simulink model "PenduloDoblesimulink"  (R2024a)
settings: Solver=VariableStepAuto  StartTime=0.0  StopTime=10.0  RelTol=1e-3
settings Model: Creator=hmax6  LastModifiedBy=100117273
settings RTWCC: GPUComputeCapability=3.5

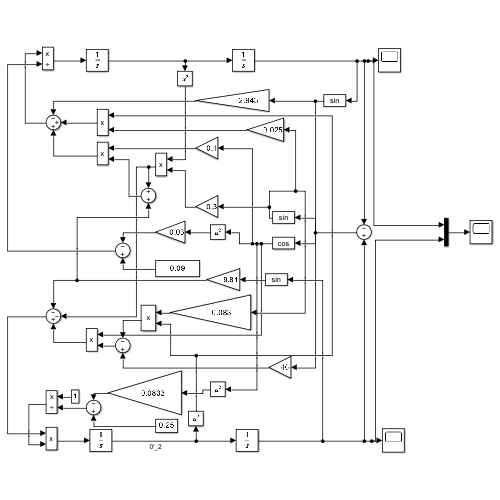
[thumbnail: Simulink's stored preview of the top-level diagram]
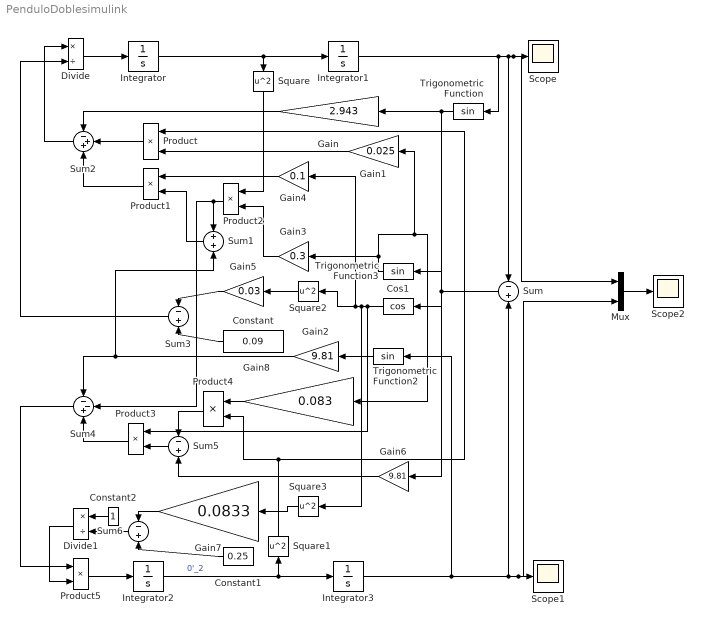
== system PenduloDoblesimulink ==
  Constant : Constant  Value=0.09
  Constant1 : Constant  Value=0.25
  Constant2 : Constant
  Cos1 : Trigonometry  Operator=cos
  Divide : Product  Inputs=*/
  Divide1 : Product  Inputs=*/
  Gain : Gain  Gain=2.943
  Gain1 : Gain  Gain=0.025
  Gain2 : Gain  Gain=9.81
  Gain3 : Gain  Gain=0.3
  Gain4 : Gain  Gain=0.1
  Gain5 : Gain  Gain=0.03
  Gain6 : Gain  Gain=9.81
  Gain7 : Gain  Gain=0.0833
  Gain8 : Gain  Gain=0.083
  Integrator : Integrator
  Integrator1 : Integrator
  Integrator2 : Integrator
  Integrator3 : Integrator  InitialCondition=0.35
  Mux : Mux  Inputs=2
  Product{,1..5} (6 alike) : Product
  Scope : Scope
  Scope1 : Scope
  Scope2 : Scope
  Square{,1..3} (4 alike) : Math  Operator=square
  Sum{,3,5..6} (4 alike) : Sum  Inputs=-+
  Sum1 : Sum
  Sum2 : Sum  Inputs=-++
  Sum4 : Sum  Inputs=--+
  Trigonometric Function : Trigonometry
  Trigonometric Function2 : Trigonometry
  Trigonometric Function3 : Trigonometry
  wires:
  Constant/1 -> Sum3/2
  Sum3/1 -> Divide/2
  Square/1 -> Product2/1
  Product3/1 -> Sum4/3
  Product2/1 -> Sum4/2, Sum1/1
  Gain7/1 -> Sum6/1
  Sum1/1 -> Product1/2
  Gain2/1 -> Sum4/1, Sum1/2
  Product/1 -> Sum2/2
  Gain/1 -> Sum2/1
  Square1/1 -> Product/1, Product4/2
  Integrator/1 -> Integrator1/1, Square/1
  Gain1/1 -> Product/2
  Integrator1/1 -> Mux/1, Scope/1, Sum/1, Trigonometric Function/1
  Product1/1 -> Sum2/3
  Trigonometric Function3/1 -> Gain8/1, Gain1/1, Gain3/1
  Cos1/1 -> Gain4/1, Square2/1, Square3/1, Product3/1
  Mux/1 -> Scope2/1
  Trigonometric Function/1 -> Gain/1, Gain6/1
  Square3/1 -> Gain7/1
  Sum2/1 -> Divide/1
  Integrator2/1 -> Integrator3/1, Square1/1  "0'_2"
  Sum/1 -> Trigonometric Function3/1, Cos1/1
  Trigonometric Function2/1 -> Gain2/1
  Product4/1 -> Sum5/1
  Divide1/1 -> Product5/2
  Sum6/1 -> Divide1/2
  Gain8/1 -> Product4/1
  Integrator3/1 -> Mux/2, Scope1/1, Sum/2, Trigonometric Function2/1
  Constant2/1 -> Divide1/1
  Constant1/1 -> Sum6/2
  Divide/1 -> Integrator/1
  Square2/1 -> Gain5/1
  Gain3/1 -> Product2/2
  Sum4/1 -> Product5/1
  Product5/1 -> Integrator2/1
  Gain6/1 -> Sum5/2
  Sum5/1 -> Product3/2
  Gain5/1 -> Sum3/1
  Gain4/1 -> Product1/1
